simulink model "flanger"  (R2021b)
settings: Solver=VariableStepAuto  StartTime=0.0  StopTime=20  RelTol=1e-3
libraries: dspsrcs4 x1
settings Model: Creator=holde  LastModifiedBy=holde

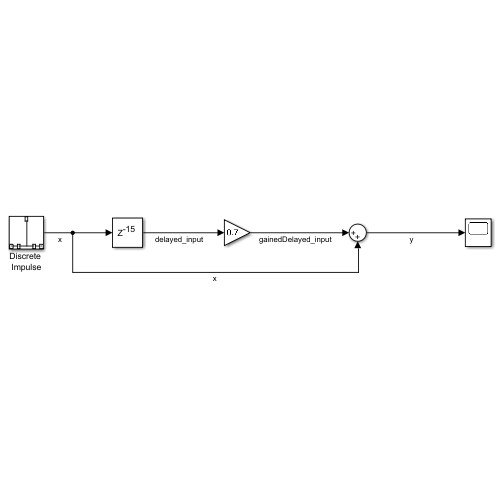
[thumbnail: Simulink's stored preview of the top-level diagram]
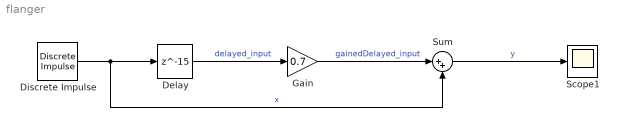
== system flanger ==
  Delay : Delay  DelayLength=15  InitialCondition=0
  Discrete Impulse : dspsrcs4/Discrete  Impulse  Delay=0  SampleTime=1  FrameSample=1  OutputFrames=off  dataType=double  isSigned=on  wordLen=16  udDataType=sfix(16)  fracBitsMode=Best precision  numFracBits=15  OutDataTypeStr=double  LastOutDataTypeStr=double
  Gain : Gain  Gain=0.7
  Scope1 : Scope
  Sum : Sum  Inputs=|++
  wires:
  Discrete Impulse/1 -> Sum/2, Delay/1  "x"
  Delay/1 -> Gain/1  "delayed_input"
  Gain/1 -> Sum/1  "gainedDelayed_input"
  Sum/1 -> Scope1/1  "y"
